simulink model "simulate_robot_and_controller2DOF"  (Simulink 9.1)
settings: Solver=ode45  StartTime=0.0  StopTime=0.6  FixedStep=0.005  RelTol=1e-3  EnableMultiTasking=on
undefined symbols (not defined in the file or in its folder): call_direct_dynamics_2dofplanar_s5b
settings Model: SuppressorTable=22 serialization::archive 11 0 6 0 0 0 0 0  Creator=arturo  LastModifiedBy=arturogilaparicio
settings DataIOCC: SignalLoggingSaveFormat=ModelDataLogs
settings OptimizationCC: ExpressionDepthLimit=2147483647
settings DebuggingCC: SolverPrmCheckMsg=warning  FcnCallInpInsideContextMsg=warning  StateNameClashWarn=warning
settings SFSimCC: SimParseCustomCode=off
settings GRTTargetCC: GeneratePreprocessorConditionals=Disable all

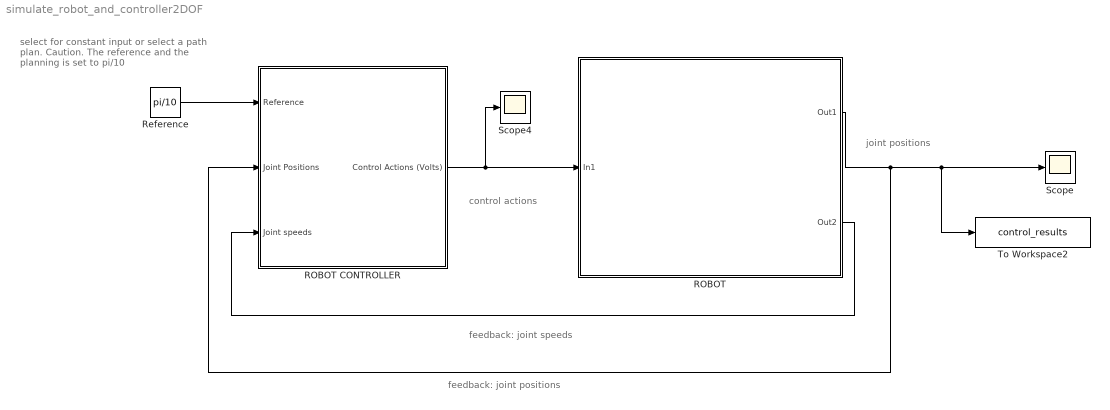
== system simulate_robot_and_controller2DOF ==
  note: select for constant input or select
      | a path plan. Caution. The reference and
      | the planning is set to pi/10
  note: control actions
  note: feedback: joint positions
  note: joint positions
  note: feedback: joint speeds
  ROBOT : Subsystem
      mask Display: image(imread('images/robot2dof.png'))
  ROBOT CONTROLLER : Subsystem  Description=ROBOT CONTROLLER
      mask Display: image(imread('images/robot-controller.jpg'))
  Reference : Constant  Value=pi/10
  Scope : Scope
  Scope4 : Scope
  To Workspace2 : ToWorkspace  VariableName=control_results  SampleTime=-1
  wires:
  ROBOT CONTROLLER/1(Control Actions (Volts)) -> ROBOT/1(In1), Scope4/1
  ROBOT/1(Out1) -> To Workspace2/1, Scope/1, ROBOT CONTROLLER/2(Joint Positions)
  Reference/1 -> ROBOT CONTROLLER/1(Reference)
  ROBOT/2(Out2) -> ROBOT CONTROLLER/3(Joint speeds)

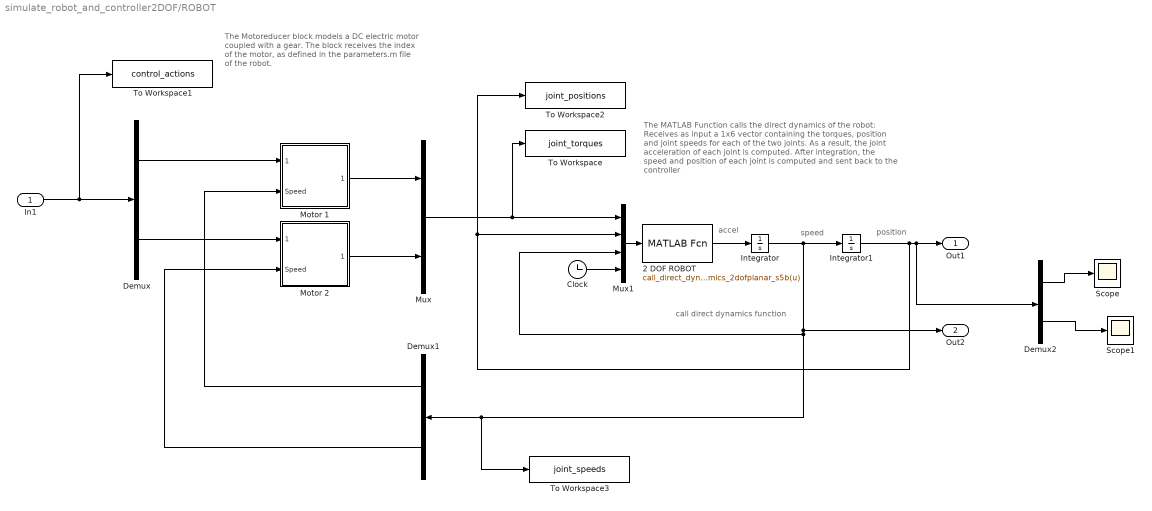
== system simulate_robot_and_controller2DOF/ROBOT ==
  note: accel
  note: speed
  note: position
  note: The MATLAB Function calls the direct dynamics of the robot:
      | Receives as input a 1x6 vector containing the
      | torques, position and joint
      | speeds for each of the two joints. As a result, the joint
      | acceleration of each joint is computed.
      | After integration, the speed and position of each joint
      | is computed and sent back to the controller
  note: call direct dynamics
      |  function
  note: The Motoreducer block models a DC
      | electric motor coupled with a gear.
      | The block receives the index of the motor,
      | as defined in the parameters.m file of the robot.
  In1 : Inport
  2 DOF ROBOT : MATLABFcn  MATLABFcn=call_direct_dynamics_2dofplanar_s5b(u)  OutputDimensions=2
  Clock : Clock
  Demux : Demux  Outputs=2
  Demux1 : Demux  Outputs=2
  Demux2 : Demux  Outputs=2
  Integrator : Integrator  InitialCondition=[0 0 ]
  Integrator1 : Integrator  InitialCondition=[0 0]
  Motor 1 : Subsystem
  Motor 2 : Subsystem
  Mux : Mux  Inputs=2
  Mux1 : Mux
  Scope : Scope
  Scope1 : Scope
  To Workspace : ToWorkspace  VariableName=joint_torques  SampleTime=-1
  To Workspace1 : ToWorkspace  VariableName=control_actions  SampleTime=-1
  To Workspace2 : ToWorkspace  VariableName=joint_positions  SampleTime=-1
  To Workspace3 : ToWorkspace  VariableName=joint_speeds  SampleTime=-1
  Out1 : Outport
  Out2 : Outport  Port=2
  wires:
  Demux/1 -> Motor 1/1(Input (Volts))
  Demux/2 -> Motor 2/1(Input (Volts))
  Mux1/1 -> 2 DOF ROBOT/1
  2 DOF ROBOT/1 -> Integrator/1
  Motor 1/1(Output Torque) -> Mux/1
  Demux1/1 -> Motor 1/2(Speed)
  Motor 2/1(Output Torque) -> Mux/2
  Demux1/2 -> Motor 2/2(Speed)
  In1/1 -> To Workspace1/1, Demux/1
  Mux/1 -> Mux1/1, To Workspace/1
  Clock/1 -> Mux1/4
  Integrator/1 -> Integrator1/1, To Workspace3/1, Demux1/1, Mux1/3, Out2/1
  Integrator1/1 -> Demux2/1, Out1/1, Mux1/2, To Workspace2/1
  Demux2/1 -> Scope/1
  Demux2/2 -> Scope1/1

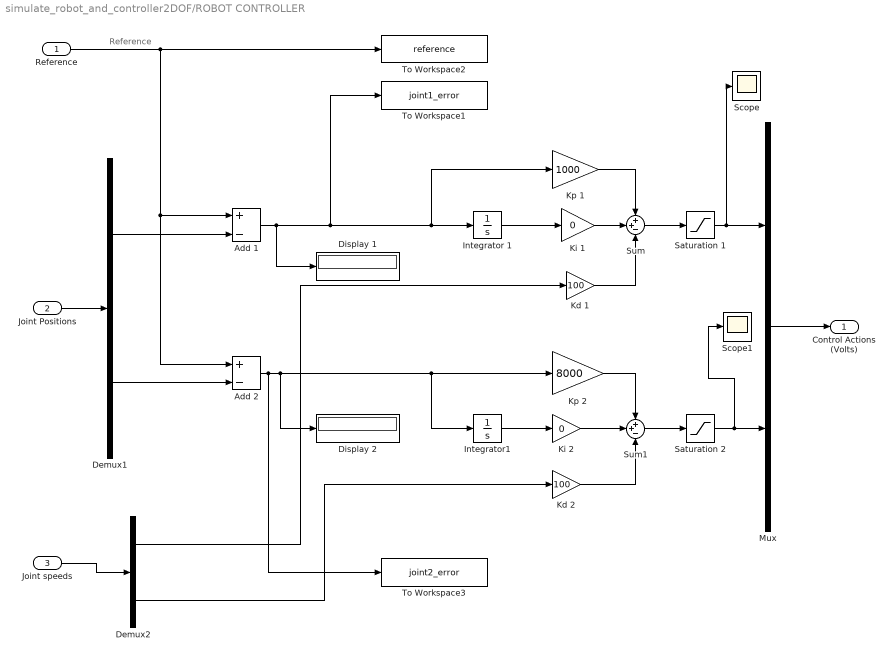
== system simulate_robot_and_controller2DOF/ROBOT CONTROLLER ==
  note: Reference
  Reference : Inport
  Joint Positions : Inport  Port=2
  Joint speeds : Inport  Port=3
  Add 1 : Sum  Inputs=+-
  Add 2 : Sum  Inputs=+-
  Demux1 : Demux  Outputs=2
  Demux2 : Demux  Outputs=2
  Display 1 : Display
  Display 2 : Display
  Integrator 1 : Integrator
  Integrator1 : Integrator
  Kd 1 : Gain  Gain=100
  Kd 2 : Gain  Gain=100
  Ki 1 : Gain  Gain=0
  Ki 2 : Gain  Gain=0
  Kp 1 : Gain  Gain=1000
  Kp 2 : Gain  Gain=8000
  Mux : Mux  Inputs=2
  Saturation 1 : Saturate  UpperLimit=100  LowerLimit=-100  ZeroCross=off
  Saturation 2 : Saturate  UpperLimit=100  LowerLimit=-100  ZeroCross=off
  Scope : Scope
  Scope1 : Scope
  Sum : Sum  Inputs=++-
  Sum1 : Sum  Inputs=++-
  To Workspace1 : ToWorkspace  VariableName=joint1_error  SampleTime=-1
  To Workspace2 : ToWorkspace  VariableName=reference  SampleTime=-1
  To Workspace3 : ToWorkspace  VariableName=joint2_error  SampleTime=-1
  Control Actions (Volts) : Outport
  wires:
  Sum/1 -> Saturation 1/1
  Mux/1 -> Control Actions (Volts)/1
  Demux1/2 -> Add 2/2
  Demux1/1 -> Add 1/2
  Reference/1 -> To Workspace2/1, Add 1/1, Add 2/1
  Add 2/1 -> To Workspace3/1, Display 2/1, Integrator1/1, Kp 2/1
  Saturation 1/1 -> Scope/1, Mux/1
  Saturation 2/1 -> Scope1/1, Mux/2
  Integrator 1/1 -> Ki 1/1
  Demux2/1 -> Kd 1/1
  Kp 1/1 -> Sum/1
  Ki 1/1 -> Sum/2
  Kd 1/1 -> Sum/3
  Add 1/1 -> Display 1/1, To Workspace1/1, Integrator 1/1, Kp 1/1
  Sum1/1 -> Saturation 2/1
  Integrator1/1 -> Ki 2/1
  Demux2/2 -> Kd 2/1
  Kp 2/1 -> Sum1/1
  Ki 2/1 -> Sum1/2
  Kd 2/1 -> Sum1/3
  Joint Positions/1 -> Demux1/1
  Joint speeds/1 -> Demux2/1

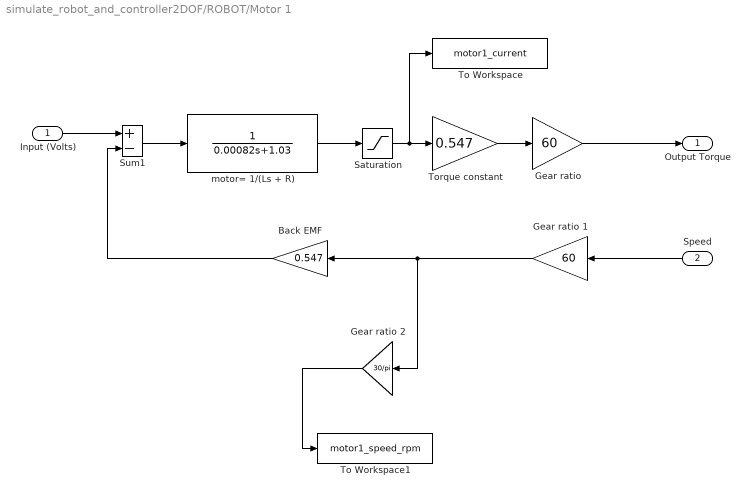
== system simulate_robot_and_controller2DOF/ROBOT/Motor 1 ==
  Input (Volts) : Inport
  Speed : Inport  Port=2
  Back EMF : Gain  Gain=0.547  SaturateOnIntegerOverflow=on  OutDataTypeStr=Inherit: Same as input  ParamDataTypeStr=Inherit: Same as input
  Gear ratio : Gain  Gain=60  SaturateOnIntegerOverflow=on  OutDataTypeStr=Inherit: Same as input  ParamDataTypeStr=Inherit: Same as input
  Gear ratio 1 : Gain  Gain=60  SaturateOnIntegerOverflow=on  OutDataTypeStr=Inherit: Same as input  ParamDataTypeStr=Inherit: Same as input
  Gear ratio 2 : Gain  Gain=30/pi  SaturateOnIntegerOverflow=on  OutDataTypeStr=Inherit: Same as input  ParamDataTypeStr=Inherit: Same as input
  Saturation : Saturate  UpperLimit=30  LowerLimit=-30  ZeroCross=off
  Sum1 : Sum  Inputs=+-  SaturateOnIntegerOverflow=on  InputSameDT=on  OutDataTypeStr=Inherit: Same as first input
  To Workspace : ToWorkspace  VariableName=motor1_current  SampleTime=-1
  To Workspace1 : ToWorkspace  VariableName=motor1_speed_rpm  SampleTime=-1
  Torque constant : Gain  Gain=0.547  SaturateOnIntegerOverflow=on  OutDataTypeStr=Inherit: Same as input  ParamDataTypeStr=Inherit: Same as input
  motor= 1/(Ls + R) : TransferFcn  Denominator=[0.00082 1.03]
  Output Torque : Outport  InitialOutput=0
  wires:
  Speed/1 -> Gear ratio 1/1
  Input (Volts)/1 -> Sum1/1
  Back EMF/1 -> Sum1/2
  Sum1/1 -> motor= 1/(Ls + R)/1
  Gear ratio/1 -> Output Torque/1
  Torque constant/1 -> Gear ratio/1
  motor= 1/(Ls + R)/1 -> Saturation/1
  Saturation/1 -> To Workspace/1, Torque constant/1
  Gear ratio 2/1 -> To Workspace1/1
  Gear ratio 1/1 -> Gear ratio 2/1, Back EMF/1

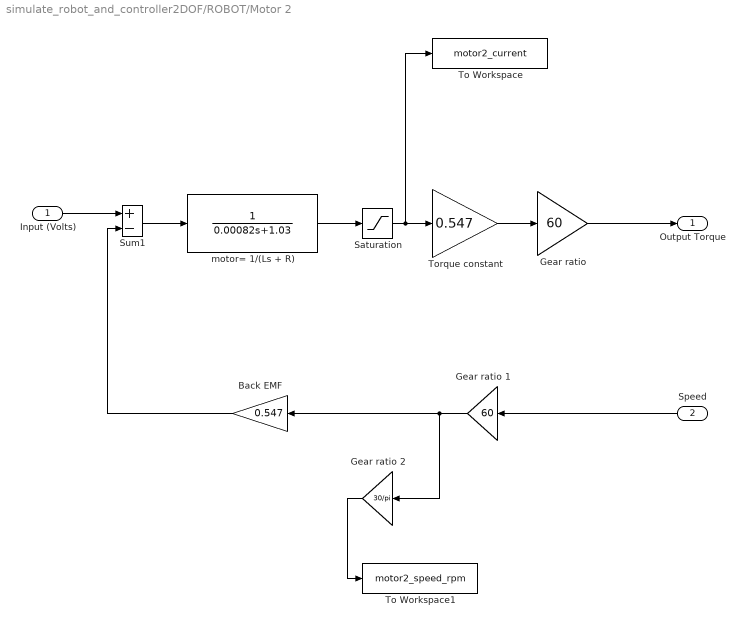
== system simulate_robot_and_controller2DOF/ROBOT/Motor 2 ==
  Input (Volts) : Inport
  Speed : Inport  Port=2
  Back EMF : Gain  Gain=0.547  SaturateOnIntegerOverflow=on  OutDataTypeStr=Inherit: Same as input  ParamDataTypeStr=Inherit: Same as input
  Gear ratio : Gain  Gain=60  SaturateOnIntegerOverflow=on  OutDataTypeStr=Inherit: Same as input  ParamDataTypeStr=Inherit: Same as input
  Gear ratio 1 : Gain  Gain=60  SaturateOnIntegerOverflow=on  OutDataTypeStr=Inherit: Same as input  ParamDataTypeStr=Inherit: Same as input
  Gear ratio 2 : Gain  Gain=30/pi  SaturateOnIntegerOverflow=on  OutDataTypeStr=Inherit: Same as input  ParamDataTypeStr=Inherit: Same as input
  Saturation : Saturate  UpperLimit=30  LowerLimit=-30  ZeroCross=off
  Sum1 : Sum  Inputs=+-  SaturateOnIntegerOverflow=on  InputSameDT=on  OutDataTypeStr=Inherit: Same as first input
  To Workspace : ToWorkspace  VariableName=motor2_current  SampleTime=-1
  To Workspace1 : ToWorkspace  VariableName=motor2_speed_rpm  SampleTime=-1
  Torque constant : Gain  Gain=0.547  SaturateOnIntegerOverflow=on  OutDataTypeStr=Inherit: Same as input  ParamDataTypeStr=Inherit: Same as input
  motor= 1/(Ls + R) : TransferFcn  Denominator=[0.00082 1.03]
  Output Torque : Outport  InitialOutput=0
  wires:
  Saturation/1 -> To Workspace/1, Torque constant/1
  motor= 1/(Ls + R)/1 -> Saturation/1
  Torque constant/1 -> Gear ratio/1
  Gear ratio/1 -> Output Torque/1
  Sum1/1 -> motor= 1/(Ls + R)/1
  Back EMF/1 -> Sum1/2
  Input (Volts)/1 -> Sum1/1
  Speed/1 -> Gear ratio 1/1
  Gear ratio 1/1 -> Gear ratio 2/1, Back EMF/1
  Gear ratio 2/1 -> To Workspace1/1
